simulink model "Rail_CtlLoopLimMeUn"  (R2016b)
settings: configuration reference "CodeGenConfigSet" (kept outside this file)
values from neighbouring files (symbols this model uses):
  Rail_dvolMeUnCtlUpLim_C = Calibration.Parameter    [init_Rail_CtlLoopLimMeUn.m]
  Rail_dvolMeUnCtlUpLim_CUR = Calibration.Parameter    [init_Rail_CtlLoopLimMeUn.m]
  Rail_dvolMeUnCtlUpLim_CURX = Calibration.Parameter    [init_Rail_CtlLoopLimMeUn.m]
settings Model: Creator=lenovo  LastModifiedBy=wangrui
settings ConfigSetRef: SourceLocation=Base Workspace

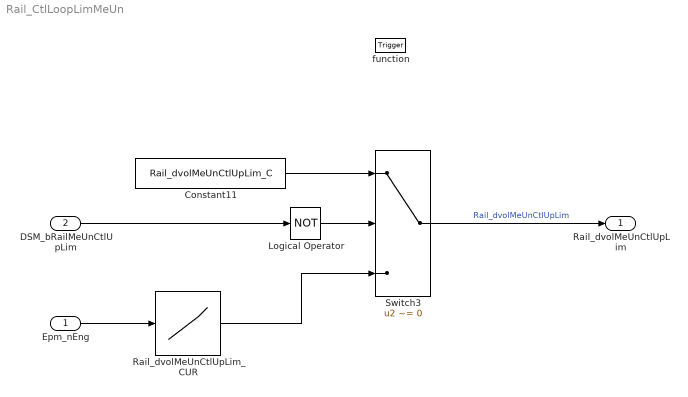
== system Rail_CtlLoopLimMeUn ==
  Epm_nEng : Inport  Tag=rpm  Description=Engine speed  OutMin=0  OutMax=6000  OutDataTypeStr=EngSpeed_rpm
  DSM_bRailMeUnCtlUpLim : Inport  Description=state of FId_Rail_MeUnCtlUpLim  Port=2  OutMin=0  OutMax=1  OutDataTypeStr=boolean
  function : TriggerPort  TriggerType=function-call  VariantControl=Variant
  Constant11 : Constant  Value=Rail_dvolMeUnCtlUpLim_C  SampleTime=-1
  Logical Operator : Logic  Operator=NOT  Inputs=1  AllPortsSameDT=off  OutDataTypeStr=boolean
  Rail_dvolMeUnCtlUpLim_CUR : Lookup_n-D  NumberOfTableDimensions=1  BreakpointsForDimension1=Rail_dvolMeUnCtlUpLim_CURX  IndexSearchMethod=Linear search  BeginIndexSearchUsingPreviousIndexResult=on  Table=Rail_dvolMeUnCtlUpLim_CUR  ExtrapMethod=Clip  UseLastTableValue=on  InternalRulePriority=Speed  OutDataTypeStr=Inherit: Inherit via back propagation  SaturateOnIntegerOverflow=on
  Switch3 : Switch  Criteria=u2 ~= 0  InputSameDT=on
  Rail_dvolMeUnCtlUpLim : Outport  Tag=mm^3/s  Description=Upper actuator value limit for pressure governing by metering unit  OutMin=0  OutMax=327670  OutDataTypeStr=FuelVol_mm3_s
  wires:
  Switch3/1 -> Rail_dvolMeUnCtlUpLim/1  "Rail_dvolMeUnCtlUpLim"
  Rail_dvolMeUnCtlUpLim_CUR/1 -> Switch3/3
  Logical Operator/1 -> Switch3/2
  Constant11/1 -> Switch3/1
  DSM_bRailMeUnCtlUpLim/1 -> Logical Operator/1
  Epm_nEng/1 -> Rail_dvolMeUnCtlUpLim_CUR/1
